simulink model "projectunfoldparallel"  (R2015b)
settings: Solver=FixedStepDiscrete  SolverMode=SingleTasking  StartTime=0.0  StopTime=10.0  RelTol=1e-3
libraries: shlslibv1 x387
settings Model: synDspstartup=OK  Creator=sdatta24  LastModifiedBy=agill17
settings DataIOCC: SaveOutput=off  SignalLogging=off  SaveTime=off
settings OptimizationCC: DefaultParameterBehavior=Inlined
settings DebuggingCC: AlgebraicLoopMsg=error  InheritedTsInSrcMsg=none

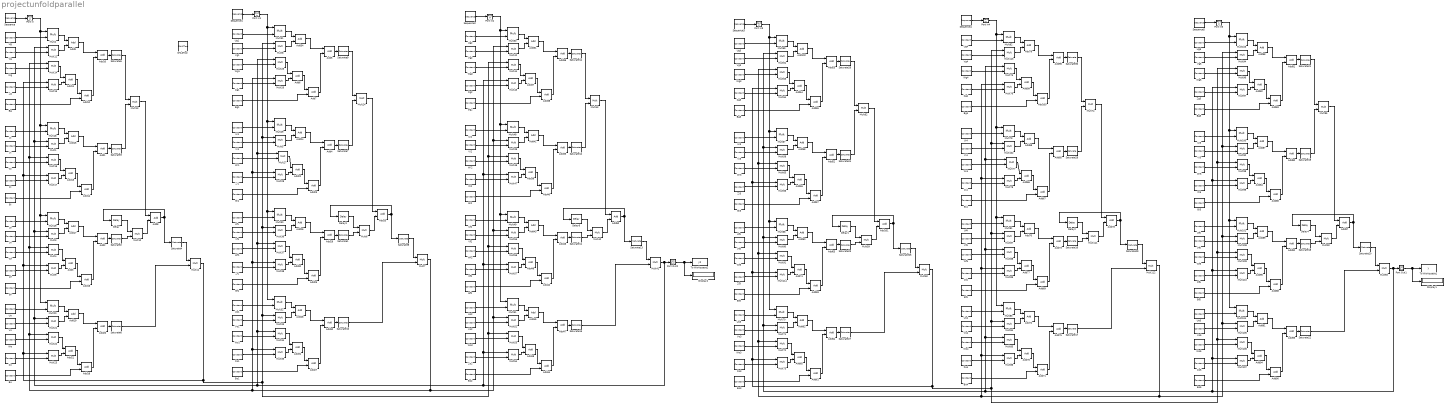
== system projectunfoldparallel ==
  Add{1..2,4..5,10,29,35..36,46,52..53,63,73,80..81,85,92,96} (18 alike) : shlslibv1/Math Functions/Add  syn_add_opr=++  syn_out_f=Full Precision  syn_out_wl=16  syn_out_fl=8  syn_out_dt=signed  syn_out_sat=off  syn_out_rnd=Floor (Truncate)  synBlockType=primitive  synLatency=0  synBlockId=96  syn_sum_of_rows=off  syn_inh_port=off  syn_inh_st=on  syn_inh_stf=1  syn_en_pipe=off  syn_pipe_stg=syn_max_pipeline  syn_flow_ctrl=off
  Add{3,6..8,11..14,16,18,21..23,25,27,31..33,37..40,42,44,48..50,54..57,59,61,65..67,69,71,74,76..78,82..84,86,88,90,94..95,97,99..101} (54 alike) : shlslibv1/Math Functions/Add  syn_add_opr=++  syn_out_f=Specify  syn_out_wl=25  syn_out_fl=7  syn_out_dt=unsigned  syn_out_sat=off  syn_out_rnd=Floor (Truncate)  synBlockType=primitive  synLatency=0  synBlockId=96  syn_sum_of_rows=off  syn_inh_port=off  syn_inh_st=on  syn_inh_stf=1  syn_en_pipe=off  syn_pipe_stg=syn_max_pipeline  syn_flow_ctrl=off
  Add{9,15,17,19,24,26,28,34,41,43,45,51,58,60,62,68,70,72,79,87,89,91,98,102} (24 alike) : shlslibv1/Math Functions/Add  syn_add_opr=++  syn_out_f=Specify  syn_out_wl=25  syn_out_fl=7  syn_out_dt=unsigned  syn_out_sat=off  syn_out_rnd=Floor (Truncate)  synBlockType=primitive  synLatency=0  synBlockId=96  syn_sum_of_rows=off  syn_inh_port=off  syn_inh_st=on  syn_inh_stf=1  syn_en_pipe=on  syn_pipe_stg=2  syn_flow_ctrl=off
  Add{20,30,47,64,75,93} (6 alike) : shlslibv1/Math Functions/Add  syn_add_opr=++  syn_out_f=Full Precision  syn_out_wl=16  syn_out_fl=8  syn_out_dt=signed  syn_out_sat=off  syn_out_rnd=Floor (Truncate)  synBlockType=primitive  synLatency=0  synBlockId=96  syn_sum_of_rows=off  syn_inh_port=off  syn_inh_st=on  syn_inh_stf=1  syn_en_pipe=on  syn_pipe_stg=4  syn_flow_ctrl=off
  Bf{,1..5} (6 alike) : shlslibv1/Sources/Constant  syn_cst_val=1  syn_cst_format=Specify  syn_cst_wl=25  syn_cst_fl=7  syn_cst_dt=unsigned  syn_cst_rnd=on  syn_cst_st=1/300e6  synBlockType=primitive  synLatency=0  synBlockId=15
  Bg{,1..5} (6 alike) : shlslibv1/Sources/Constant  syn_cst_val=1  syn_cst_format=Specify  syn_cst_wl=25  syn_cst_fl=7  syn_cst_dt=unsigned  syn_cst_rnd=on  syn_cst_st=1/300e6  synBlockType=primitive  synLatency=0  synBlockId=15
  Bi{,1..5} (6 alike) : shlslibv1/Sources/Constant  syn_cst_val=1  syn_cst_format=Specify  syn_cst_wl=25  syn_cst_fl=7  syn_cst_dt=unsigned  syn_cst_rnd=on  syn_cst_st=1/300e6  synBlockType=primitive  synLatency=0  synBlockId=15
  Bo{,1..5} (6 alike) : shlslibv1/Sources/Constant  syn_cst_val=1  syn_cst_format=Specify  syn_cst_wl=25  syn_cst_fl=7  syn_cst_dt=unsigned  syn_cst_rnd=on  syn_cst_st=1/300e6  synBlockType=primitive  synLatency=0  synBlockId=15
  Delay{,1..4,6} (6 alike) : shlslibv1/Memories/Delay  syn_delay_val=1  synBlockType=primitive  synLatency=1  synBlockId=104
  Display1 : Display
  Display2 : Display
  Mult{1..114} (114 alike) : shlslibv1/Math Functions/Mult  syn_out_f=Specify  syn_out_wl=25  syn_out_fl=7  syn_out_dt=unsigned  syn_out_sat=off  syn_out_rnd=Floor (Truncate)  syn_inh_port=off  syn_inh_st=off  syn_inh_stf=1  syn_en_pipe=off  syn_pipe_stg=syn_max_pipeline  syn_flow_ctrl=off  synBlockType=primitive  synLatency=0  synBlockId=3  syn_opr_mode=1
  Port In{,1..5} (6 alike) : shlslibv1/Ports & Subsystems/Port In  syn_out_wl=25  syn_out_fl=7  syn_out_dt=unsigned  syn_out_st=1/300e6  syn_capture=on  syn_register=on  syn_out_sat=off  syn_out_rnd=on  synBlockType=port  synLatency=1  synBlockId=0
  Port Out1 : shlslibv1/Ports & Subsystems/Port Out  syn_capture=on  syn_register=on  synBlockType=port  synLatency=1  synBlockId=1
  Port Out2 : shlslibv1/Ports & Subsystems/Port Out  syn_capture=on  syn_register=on  synBlockType=port  synLatency=1  synBlockId=1
  SHLSTool : shlslibv1/SHLSTool  synBlockType=tool  syn_dsp_mode=FPGA
  Saturate{1..3,6..7,10..12,15..19,22..24,27..28} (18 alike) : shlslibv1/Signal Operations/Saturate  syn_sat_mode=Constant  syn_pos_val=1  syn_neg_val=0  syn_sat_fl=7  syn_sat_rnd=on  syn_out_f=Same as Input  syn_out_wl=16  syn_out_fl=15  syn_out_dt=signed  syn_out_rnd=on  syn_pipe=on  syn_sat_ind=off  synBlockType=custom  synLatency=1
  Saturate{4..5,8..9,13..14,20..21,25..26,29..30} (12 alike) : shlslibv1/Signal Operations/Saturate  syn_sat_mode=Constant  syn_pos_val=1  syn_neg_val=-1  syn_sat_fl=7  syn_sat_rnd=on  syn_out_f=Same as Input  syn_out_wl=16  syn_out_fl=15  syn_out_dt=signed  syn_out_rnd=on  syn_pipe=on  syn_sat_ind=off  synBlockType=custom  synLatency=1
  Sequence{,1..5} (6 alike) : shlslibv1/Sources/Sequence  syn_seq_vec=[100 100 100 100 100 100 100 100 100 200 200 200 200 200 200 200 200 200 300 300 300 300 300 300 300 300 300 400 400 400 400 400 400 400 400 400 500 500 500 500 500 500 500 500 500 600 600 600 600 600 600 600 600 600 700 700 700 700 700 700 700 700 700 800 800 800 800 800 800 800 800 800 900 900 900 900 900 900 900 900 900]  syn_seq_wl=25  syn_seq_fl=7  syn_seq_dt=unsigned  syn_rst_port=off  syn_en_port=off  syn_seq_st=1/300e6  synBlockType=custom  synLatency=1
  To Workspace1 : ToWorkspace  VariableName=y  SaveFormat=Structure With Time  SampleTime=1/300e6
  To Workspace2 : ToWorkspace  VariableName=y2  SaveFormat=Structure With Time  SampleTime=1/300e6
  Uf{,1..5} (6 alike) : shlslibv1/Sources/Constant  syn_cst_val=0  syn_cst_format=Specify  syn_cst_wl=25  syn_cst_fl=7  syn_cst_dt=unsigned  syn_cst_rnd=on  syn_cst_st=1/300e6  synBlockType=primitive  synLatency=0  synBlockId=15
  Ug{,1..5} (6 alike) : shlslibv1/Sources/Constant  syn_cst_val=1  syn_cst_format=Specify  syn_cst_wl=25  syn_cst_fl=7  syn_cst_dt=unsigned  syn_cst_rnd=on  syn_cst_st=1/300e6  synBlockType=primitive  synLatency=0  synBlockId=15
  Ui{,1..5} (6 alike) : shlslibv1/Sources/Constant  syn_cst_val=1  syn_cst_format=Specify  syn_cst_wl=25  syn_cst_fl=7  syn_cst_dt=unsigned  syn_cst_rnd=on  syn_cst_st=1/300e6  synBlockType=primitive  synLatency=0  synBlockId=15
  Uo{,1..5} (6 alike) : shlslibv1/Sources/Constant  syn_cst_val=1  syn_cst_format=Specify  syn_cst_wl=25  syn_cst_fl=7  syn_cst_dt=unsigned  syn_cst_rnd=on  syn_cst_st=1/300e6  synBlockType=primitive  synLatency=0  synBlockId=15
  Vf{,1..5} (6 alike) : shlslibv1/Sources/Constant  syn_cst_val=0  syn_cst_format=Specify  syn_cst_wl=25  syn_cst_fl=7  syn_cst_dt=unsigned  syn_cst_rnd=on  syn_cst_st=1/300e6  synBlockType=primitive  synLatency=0  synBlockId=15
  Vg{,1..5} (6 alike) : shlslibv1/Sources/Constant  syn_cst_val=1  syn_cst_format=Specify  syn_cst_wl=25  syn_cst_fl=7  syn_cst_dt=unsigned  syn_cst_rnd=on  syn_cst_st=1/300e6  synBlockType=primitive  synLatency=0  synBlockId=15
  Vi{,1..5} (6 alike) : shlslibv1/Sources/Constant  syn_cst_val=1  syn_cst_format=Specify  syn_cst_wl=25  syn_cst_fl=7  syn_cst_dt=unsigned  syn_cst_rnd=on  syn_cst_st=1/300e6  synBlockType=primitive  synLatency=0  synBlockId=15
  Vo{,1..5} (6 alike) : shlslibv1/Sources/Constant  syn_cst_val=1  syn_cst_format=Specify  syn_cst_wl=25  syn_cst_fl=7  syn_cst_dt=unsigned  syn_cst_rnd=on  syn_cst_st=1/300e6  synBlockType=primitive  synLatency=0  synBlockId=15
  Wf{,1..5} (6 alike) : shlslibv1/Sources/Constant  syn_cst_val=0  syn_cst_format=Specify  syn_cst_wl=25  syn_cst_fl=7  syn_cst_dt=unsigned  syn_cst_rnd=on  syn_cst_st=1/300e6  synBlockType=primitive  synLatency=0  synBlockId=15
  Wg{,1..5} (6 alike) : shlslibv1/Sources/Constant  syn_cst_val=1  syn_cst_format=Specify  syn_cst_wl=25  syn_cst_fl=7  syn_cst_dt=unsigned  syn_cst_rnd=on  syn_cst_st=1/300e6  synBlockType=primitive  synLatency=0  synBlockId=15
  Wi{,1..5} (6 alike) : shlslibv1/Sources/Constant  syn_cst_val=1  syn_cst_format=Specify  syn_cst_wl=25  syn_cst_fl=7  syn_cst_dt=unsigned  syn_cst_rnd=on  syn_cst_st=1/300e6  synBlockType=primitive  synLatency=0  synBlockId=15
  Wo{,1..5} (6 alike) : shlslibv1/Sources/Constant  syn_cst_val=1  syn_cst_format=Specify  syn_cst_wl=25  syn_cst_fl=7  syn_cst_dt=unsigned  syn_cst_rnd=on  syn_cst_st=1/300e6  synBlockType=primitive  synLatency=0  synBlockId=15
  Zf{,1..5} (6 alike) : shlslibv1/Sources/Constant  syn_cst_val=0  syn_cst_format=Specify  syn_cst_wl=25  syn_cst_fl=7  syn_cst_dt=unsigned  syn_cst_rnd=on  syn_cst_st=1/300e6  synBlockType=primitive  synLatency=0  synBlockId=15
  Zg{,1..5} (6 alike) : shlslibv1/Sources/Constant  syn_cst_val=1  syn_cst_format=Specify  syn_cst_wl=25  syn_cst_fl=7  syn_cst_dt=unsigned  syn_cst_rnd=on  syn_cst_st=1/300e6  synBlockType=primitive  synLatency=0  synBlockId=15
  Zi{,1..5} (6 alike) : shlslibv1/Sources/Constant  syn_cst_val=1  syn_cst_format=Specify  syn_cst_wl=25  syn_cst_fl=7  syn_cst_dt=unsigned  syn_cst_rnd=on  syn_cst_st=1/300e6  synBlockType=primitive  synLatency=0  synBlockId=15
  Zo{,1..5} (6 alike) : shlslibv1/Sources/Constant  syn_cst_val=1  syn_cst_format=Specify  syn_cst_wl=25  syn_cst_fl=7  syn_cst_dt=unsigned  syn_cst_rnd=on  syn_cst_st=1/300e6  synBlockType=primitive  synLatency=0  synBlockId=15
  wires:
  Sequence/1 -> Port In/1
  Ug/1 -> Mult2/2
  Vg/1 -> Mult12/2
  Mult2/1 -> Add9/1
  Mult12/1 -> Add9/2
  Add9/1 -> Add10/1
  Add10/1 -> Saturate5/1
  Saturate5/1 -> Mult13/1
  Wg/1 -> Mult14/2
  Zg/1 -> Mult15/2
  Mult14/1 -> Add11/1
  Mult15/1 -> Add11/2
  Add11/1 -> Add12/1
  Bg/1 -> Add12/2
  Add12/1 -> Add10/2
  Ui/1 -> Mult18/2
  Vi/1 -> Mult1/2
  Mult18/1 -> Add15/1
  Mult1/1 -> Add15/2
  Add15/1 -> Add1/1
  Add1/1 -> Saturate3/1
  Wi/1 -> Mult16/2
  Zi/1 -> Mult17/2
  Mult16/1 -> Add13/1
  Mult17/1 -> Add13/2
  Add13/1 -> Add14/1
  Bi/1 -> Add14/2
  Add14/1 -> Add1/2
  Saturate3/1 -> Mult13/2
  Uf/1 -> Mult19/2
  Vf/1 -> Mult3/2
  Mult19/1 -> Add17/1
  Mult3/1 -> Add17/2
  Add17/1 -> Add2/1
  Add2/1 -> Saturate2/1
  Wf/1 -> Mult4/2
  Zf/1 -> Mult9/2
  Mult4/1 -> Add3/1
  Mult9/1 -> Add3/2
  Add3/1 -> Add16/1
  Bf/1 -> Add16/2
  Add16/1 -> Add2/2
  Uo/1 -> Mult20/2
  Vo/1 -> Mult21/2
  Mult20/1 -> Add19/1
  Mult21/1 -> Add19/2
  Add19/1 -> Add20/1
  Add20/1 -> Saturate6/1
  Wo/1 -> Mult22/2
  Zo/1 -> Mult23/2
  Mult22/1 -> Add21/1
  Mult23/1 -> Add21/2
  Add21/1 -> Add18/1
  Bo/1 -> Add18/2
  Add18/1 -> Add20/2
  Delay/1 -> Mult10/1
  Mult10/1 -> Add8/2
  Add8/1 -> Delay/1, Saturate4/1
  Saturate4/1 -> Mult11/1
  Saturate2/1 -> Mult10/2
  Mult13/1 -> Add8/1
  Saturate6/1 -> Mult11/2
  Port In/1 -> Mult19/1, Mult20/1, Mult18/1, Mult2/1
  Sequence1/1 -> Port In1/1
  Ug1/1 -> Mult31/2
  Vg1/1 -> Mult8/2
  Mult31/1 -> Add34/1
  Mult8/1 -> Add34/2
  Add34/1 -> Add5/1
  Add5/1 -> Saturate9/1
  Saturate9/1 -> Mult24/1
  Wg1/1 -> Mult25/2
  Zg1/1 -> Mult26/2
  Mult25/1 -> Add6/1
  Mult26/1 -> Add6/2
  Add6/1 -> Add7/1
  Bg1/1 -> Add7/2
  Add7/1 -> Add5/2
  Ui1/1 -> Mult29/2
  Vi1/1 -> Mult5/2
  Mult29/1 -> Add24/1
  Mult5/1 -> Add24/2
  Add24/1 -> Add4/1
  Add4/1 -> Saturate7/1
  Wi1/1 -> Mult27/2
  Zi1/1 -> Mult28/2
  Mult27/1 -> Add22/1
  Mult28/1 -> Add22/2
  Add22/1 -> Add23/1
  Bi1/1 -> Add23/2
  Add23/1 -> Add4/2
  Saturate7/1 -> Mult24/2
  Uf1/1 -> Mult30/2
  Vf1/1 -> Mult36/2
  Mult30/1 -> Add26/1
  Mult36/1 -> Add26/2
  Add26/1 -> Add29/1
  Add29/1 -> Saturate1/1
  Wf1/1 -> Mult37/2
  Zf1/1 -> Mult38/2
  Mult37/1 -> Add32/1
  Mult38/1 -> Add32/2
  Add32/1 -> Add25/1
  Bf1/1 -> Add25/2
  Add25/1 -> Add29/2
  Uo1/1 -> Mult32/2
  Vo1/1 -> Mult33/2
  Mult32/1 -> Add28/1
  Mult33/1 -> Add28/2
  Add28/1 -> Add30/1
  Add30/1 -> Saturate10/1
  Wo1/1 -> Mult34/2
  Zo1/1 -> Mult35/2
  Mult34/1 -> Add31/1
  Mult35/1 -> Add31/2
  Add31/1 -> Add27/1
  Bo1/1 -> Add27/2
  Add27/1 -> Add30/2
  Delay3/1 -> Mult6/1
  Mult6/1 -> Add33/2
  Add33/1 -> Delay3/1, Saturate8/1
  Saturate8/1 -> Mult7/1
  Saturate1/1 -> Mult6/2
  Mult24/1 -> Add33/1
  Saturate10/1 -> Mult7/2
  Port In1/1 -> Mult30/1, Mult32/1, Mult29/1, Mult31/1
  Sequence2/1 -> Port In2/1
  Ug2/1 -> Mult50/2
  Vg2/1 -> Mult42/2
  Mult50/1 -> Add51/1
  Mult42/1 -> Add51/2
  Add51/1 -> Add36/1
  Add36/1 -> Saturate14/1
  Saturate14/1 -> Mult43/1
  Wg2/1 -> Mult44/2
  Zg2/1 -> Mult45/2
  Mult44/1 -> Add37/1
  Mult45/1 -> Add37/2
  Add37/1 -> Add38/1
  Bg2/1 -> Add38/2
  Add38/1 -> Add36/2
  Ui2/1 -> Mult48/2
  Vi2/1 -> Mult39/2
  Mult48/1 -> Add41/1
  Mult39/1 -> Add41/2
  Add41/1 -> Add35/1
  Add35/1 -> Saturate12/1
  Wi2/1 -> Mult46/2
  Zi2/1 -> Mult47/2
  Mult46/1 -> Add39/1
  Mult47/1 -> Add39/2
  Add39/1 -> Add40/1
  Bi2/1 -> Add40/2
  Add40/1 -> Add35/2
  Saturate12/1 -> Mult43/2
  Uf2/1 -> Mult49/2
  Vf2/1 -> Mult55/2
  Mult49/1 -> Add43/1
  Mult55/1 -> Add43/2
  Add43/1 -> Add46/1
  Add46/1 -> Saturate11/1
  Wf2/1 -> Mult56/2
  Zf2/1 -> Mult57/2
  Mult56/1 -> Add49/1
  Mult57/1 -> Add49/2
  Add49/1 -> Add42/1
  Bf2/1 -> Add42/2
  Add42/1 -> Add46/2
  Uo2/1 -> Mult51/2
  Vo2/1 -> Mult52/2
  Mult51/1 -> Add45/1
  Mult52/1 -> Add45/2
  Add45/1 -> Add47/1
  Add47/1 -> Saturate15/1
  Wo2/1 -> Mult53/2
  Zo2/1 -> Mult54/2
  Mult53/1 -> Add48/1
  Mult54/1 -> Add48/2
  Add48/1 -> Add44/1
  Bo2/1 -> Add44/2
  Add44/1 -> Add47/2
  Delay6/1 -> Mult40/1
  Mult40/1 -> Add50/2
  Add50/1 -> Delay6/1, Saturate13/1
  Port Out2/1 -> Display2/1, To Workspace2/1
  Saturate13/1 -> Mult41/1
  Saturate11/1 -> Mult40/2
  Mult43/1 -> Add50/1
  Saturate15/1 -> Mult41/2
  Port In2/1 -> Mult49/1, Mult51/1, Mult48/1, Mult50/1
  Mult11/1 -> Mult23/1, Mult9/1, Mult17/1, Mult15/1, Mult53/1, Mult56/1, Mult46/1, Mult44/1, Mult33/1, Mult36/1, Mult5/1, Mult8/1
  Mult41/1 -> Mult54/1, Mult57/1, Mult47/1, Mult45/1, Mult34/1, Mult37/1, Mult27/1, Mult25/1, Mult21/1, Mult3/1, Mult12/1, Mult1/1, Port Out2/1
  Mult7/1 -> Mult35/1, Mult38/1, Mult28/1, Mult26/1, Mult22/1, Mult4/1, Mult16/1, Mult14/1, Mult52/1, Mult55/1, Mult39/1, Mult42/1
  Sequence3/1 -> Port In3/1
  Ug3/1 -> Mult69/2
  Vg3/1 -> Mult61/2
  Mult69/1 -> Add102/1
  Mult61/1 -> Add102/2
  Add102/1 -> Add53/1
  Add53/1 -> Saturate26/1
  Saturate26/1 -> Mult62/1
  Wg3/1 -> Mult63/2
  Zg3/1 -> Mult64/2
  Mult63/1 -> Add54/1
  Mult64/1 -> Add54/2
  Add54/1 -> Add55/1
  Bg3/1 -> Add55/2
  Add55/1 -> Add53/2
  Ui3/1 -> Mult67/2
  Vi3/1 -> Mult58/2
  Mult67/1 -> Add58/1
  Mult58/1 -> Add58/2
  Add58/1 -> Add52/1
  Add52/1 -> Saturate24/1
  Wi3/1 -> Mult65/2
  Zi3/1 -> Mult66/2
  Mult65/1 -> Add56/1
  Mult66/1 -> Add56/2
  Add56/1 -> Add57/1
  Bi3/1 -> Add57/2
  Add57/1 -> Add52/2
  Saturate24/1 -> Mult62/2
  Uf3/1 -> Mult68/2
  Vf3/1 -> Mult80/2
  Mult68/1 -> Add60/1
  Mult80/1 -> Add60/2
  Add60/1 -> Add63/1
  Add63/1 -> Saturate23/1
  Wf3/1 -> Mult91/2
  Zf3/1 -> Mult114/2
  Mult91/1 -> Add74/1
  Mult114/1 -> Add74/2
  Add74/1 -> Add59/1
  Bf3/1 -> Add59/2
  Add59/1 -> Add63/2
  Uo3/1 -> Mult70/2
  Vo3/1 -> Mult71/2
  Mult70/1 -> Add62/1
  Mult71/1 -> Add62/2
  Add62/1 -> Add64/1
  Add64/1 -> Saturate27/1
  Wo3/1 -> Mult72/2
  Zo3/1 -> Mult73/2
  Mult72/1 -> Add65/1
  Mult73/1 -> Add65/2
  Add65/1 -> Add61/1
  Bo3/1 -> Add61/2
  Add61/1 -> Add64/2
  Delay1/1 -> Mult59/1
  Mult59/1 -> Add101/2
  Add101/1 -> Delay1/1, Saturate25/1
  Saturate25/1 -> Mult60/1
  Saturate23/1 -> Mult59/2
  Mult62/1 -> Add101/1
  Saturate27/1 -> Mult60/2
  Port In3/1 -> Mult68/1, Mult70/1, Mult67/1, Mult69/1
  Sequence4/1 -> Port In4/1
  Ug4/1 -> Mult82/2
  Vg4/1 -> Mult113/2
  Mult82/1 -> Add79/1
  Mult113/1 -> Add79/2
  Add79/1 -> Add96/1
  Add96/1 -> Saturate30/1
  Saturate30/1 -> Mult74/1
  Wg4/1 -> Mult75/2
  Zg4/1 -> Mult76/2
  Mult75/1 -> Add99/1
  Mult76/1 -> Add99/2
  Add99/1 -> Add100/1
  Bg4/1 -> Add100/2
  Add100/1 -> Add96/2
  Ui4/1 -> Mult79/2
  Vi4/1 -> Mult102/2
  Mult79/1 -> Add68/1
  Mult102/1 -> Add68/2
  Add68/1 -> Add85/1
  Add85/1 -> Saturate28/1
  Wi4/1 -> Mult77/2
  Zi4/1 -> Mult78/2
  Mult77/1 -> Add66/1
  Mult78/1 -> Add66/2
  Add66/1 -> Add67/1
  Bi4/1 -> Add67/2
  Add67/1 -> Add85/2
  Saturate28/1 -> Mult74/2
  Uf4/1 -> Mult81/2
  Vf4/1 -> Mult87/2
  Mult81/1 -> Add70/1
  Mult87/1 -> Add70/2
  Add70/1 -> Add73/1
  Add73/1 -> Saturate16/1
  Wf4/1 -> Mult88/2
  Zf4/1 -> Mult89/2
  Mult88/1 -> Add77/1
  Mult89/1 -> Add77/2
  Add77/1 -> Add69/1
  Bf4/1 -> Add69/2
  Add69/1 -> Add73/2
  Uo4/1 -> Mult83/2
  Vo4/1 -> Mult84/2
  Mult83/1 -> Add72/1
  Mult84/1 -> Add72/2
  Add72/1 -> Add75/1
  Add75/1 -> Saturate17/1
  Wo4/1 -> Mult85/2
  Zo4/1 -> Mult86/2
  Mult85/1 -> Add76/1
  Mult86/1 -> Add76/2
  Add76/1 -> Add71/1
  Bo4/1 -> Add71/2
  Add71/1 -> Add75/2
  Delay2/1 -> Mult111/1
  Mult111/1 -> Add78/2
  Add78/1 -> Delay2/1, Saturate29/1
  Saturate29/1 -> Mult112/1
  Saturate16/1 -> Mult111/2
  Mult74/1 -> Add78/1
  Saturate17/1 -> Mult112/2
  Port In4/1 -> Mult81/1, Mult83/1, Mult79/1, Mult82/1
  Sequence5/1 -> Port In5/1
  Ug5/1 -> Mult103/2
  Vg5/1 -> Mult94/2
  Mult103/1 -> Add98/1
  Mult94/1 -> Add98/2
  Add98/1 -> Add81/1
  Add81/1 -> Saturate21/1
  Saturate21/1 -> Mult95/1
  Wg5/1 -> Mult96/2
  Zg5/1 -> Mult97/2
  Mult96/1 -> Add82/1
  Mult97/1 -> Add82/2
  Add82/1 -> Add83/1
  Bg5/1 -> Add83/2
  Add83/1 -> Add81/2
  Ui5/1 -> Mult100/2
  Vi5/1 -> Mult90/2
  Mult100/1 -> Add87/1
  Mult90/1 -> Add87/2
  Add87/1 -> Add80/1
  Add80/1 -> Saturate19/1
  Wi5/1 -> Mult98/2
  Zi5/1 -> Mult99/2
  Mult98/1 -> Add84/1
  Mult99/1 -> Add84/2
  Add84/1 -> Add86/1
  Bi5/1 -> Add86/2
  Add86/1 -> Add80/2
  Saturate19/1 -> Mult95/2
  Uf5/1 -> Mult101/2
  Vf5/1 -> Mult108/2
  Mult101/1 -> Add89/1
  Mult108/1 -> Add89/2
  Add89/1 -> Add92/1
  Add92/1 -> Saturate18/1
  Wf5/1 -> Mult109/2
  Zf5/1 -> Mult110/2
  Mult109/1 -> Add95/1
  Mult110/1 -> Add95/2
  Add95/1 -> Add88/1
  Bf5/1 -> Add88/2
  Add88/1 -> Add92/2
  Uo5/1 -> Mult104/2
  Vo5/1 -> Mult105/2
  Mult104/1 -> Add91/1
  Mult105/1 -> Add91/2
  Add91/1 -> Add93/1
  Add93/1 -> Saturate22/1
  Wo5/1 -> Mult106/2
  Zo5/1 -> Mult107/2
  Mult106/1 -> Add94/1
  Mult107/1 -> Add94/2
  Add94/1 -> Add90/1
  Bo5/1 -> Add90/2
  Add90/1 -> Add93/2
  Delay4/1 -> Mult92/1
  Mult92/1 -> Add97/2
  Add97/1 -> Delay4/1, Saturate20/1
  Port Out1/1 -> Display1/1, To Workspace1/1
  Saturate20/1 -> Mult93/1
  Saturate18/1 -> Mult92/2
  Mult95/1 -> Add97/1
  Saturate22/1 -> Mult93/2
  Port In5/1 -> Mult101/1, Mult104/1, Mult100/1, Mult103/1
  Mult60/1 -> Mult73/1, Mult114/1, Mult66/1, Mult64/1, Mult106/1, Mult109/1, Mult98/1, Mult96/1, Mult84/1, Mult87/1, Mult102/1, Mult113/1
  Mult93/1 -> Mult107/1, Mult110/1, Mult99/1, Mult97/1, Mult85/1, Mult88/1, Mult77/1, Mult75/1, Mult71/1, Mult80/1, Mult61/1, Mult58/1, Port Out1/1
  Mult112/1 -> Mult86/1, Mult89/1, Mult78/1, Mult76/1, Mult72/1, Mult91/1, Mult65/1, Mult63/1, Mult105/1, Mult108/1, Mult90/1, Mult94/1
